simulink model "MODEL"  (R2015a)
settings: Solver=ode45  StartTime=0.0  StopTime=10.0  RelTol=1e-3
values from neighbouring files (symbols this model uses):
  HEIGHT = val(:,3)    [runfirst.m]
  PITCH = val(:,4)    [runfirst.m]
  TIME = linspace(1,N*H,N)    [main.m]    (also in runfirst.m = val(:,1))
  X = TURN    (= 0)    [ctrlsurf.m]    (also in runfirst.m = val(:,2))
undefined symbols (not defined in the file or in its folder): Earth, WGS84
libraries: aerolibtransform2 x1, aerolibfltsims x1
settings Model: Creator=vinay  LastModifiedBy=vinay

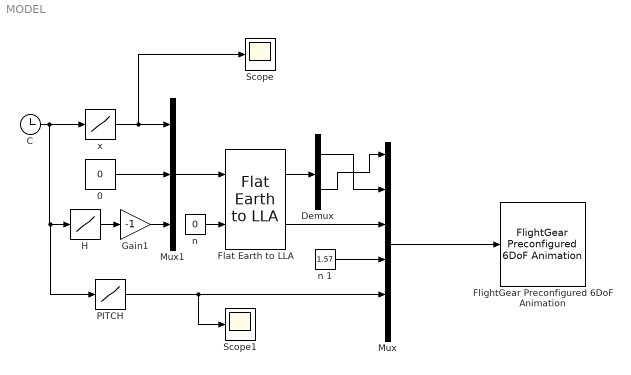
== system MODEL ==
  "0 " : Constant  Value=0
  C : Clock
  Demux : Demux  Outputs=2
  Flat Earth to LLA : aerolibtransform2/Flat Earth to LLA  units=Metric (MKS)  ptype=Earth (WGS84)  F=1/298.257223563  R=6378137  LL0=[ 34.9240 -117.8912]  psi=0
  FlightGear Preconfigured 6DoF Animation : aerolibfltsims/FlightGear Preconfigured 6DoF Animation  xFlightGearVersion=v3.0  DestinationIpAddress=127.0.0.1  DestinationPort=5502  SampleTime=1/400
  Gain1 : Gain  Gain=-1
  H : Lookup  InputValues=TIME  Table=HEIGHT  LookUpMeth=Interpolation-Use End Values  SaturateOnIntegerOverflow=on
  Mux : Mux  Inputs=6
  Mux1 : Mux  Inputs=3
  PITCH : Lookup  InputValues=TIME  Table=PITCH  LookUpMeth=Interpolation-Use End Values  SaturateOnIntegerOverflow=on
  Scope : Scope
      settings: YMin=0  YMax=25000
  Scope1 : Scope
      settings: YMin=-3.46945e-18  YMax=0.16
  "n " : Constant  Value=0
  n 1 : Constant  Value=1.57
  x : Lookup  InputValues=TIME  Table=X  LookUpMeth=Interpolation-Use End Values  SaturateOnIntegerOverflow=on
  wires:
  Mux/1 -> FlightGear Preconfigured 6DoF Animation/1
  Flat Earth to LLA/2 -> Mux/3
  Flat Earth to LLA/1 -> Demux/1
  C/1 -> H/1, PITCH/1, x/1
  PITCH/1 -> Scope1/1, Mux/5
  x/1 -> Scope/1, Mux1/1
  Mux1/1 -> Flat Earth to LLA/1
  "0 "/1 -> Mux1/2
  H/1 -> Gain1/1
  "n "/1 -> Flat Earth to LLA/2
  Gain1/1 -> Mux1/3
  Demux/1 -> Mux/2
  Demux/2 -> Mux/1
  n 1/1 -> Mux/4
